simulink model "Quarter_Car_Model_Simulation"  (R2019a)
settings: Solver=VariableStepAuto  StartTime=0.0  StopTime=16  RelTol=1e-3
settings Model: Creator=Arun  LastModifiedBy=Arun

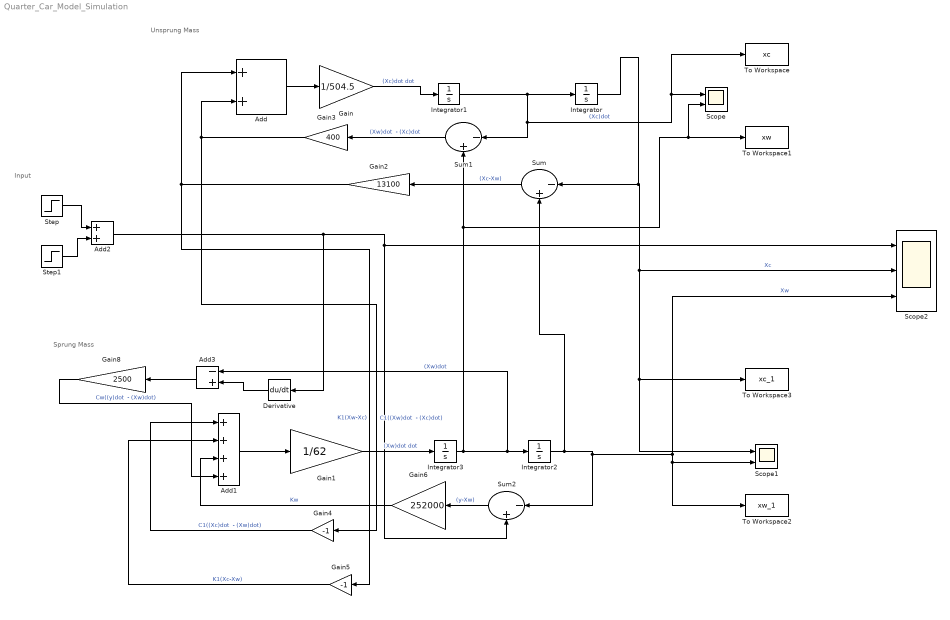
== system Quarter_Car_Model_Simulation ==
  note: Sprung Mass
  note: Unsprung Mass
  note: Input
  Add : Sum
  Add1 : Sum  Inputs=++++
  Add2 : Sum
  Add3 : Sum  Inputs=-+
  Derivative : Derivative
  Gain : Gain  Gain=1/504.5
  Gain1 : Gain  Gain=1/62
  Gain2 : Gain  Gain=13100
  Gain3 : Gain  Gain=400
  Gain4 : Gain  Gain=-1
  Gain5 : Gain  Gain=-1
  Gain6 : Gain  Gain=252000
  Gain8 : Gain  Gain=2500
  Integrator{,1..3} (4 alike) : Integrator
  Scope : Scope  NumInputPorts=2
  Scope1 : Scope  NumInputPorts=2
  Scope2 : Scope  NumInputPorts=3
  Step : Step  Time=3  After=10  SampleTime=0
  Step1 : Step  Time=5  After=-10  SampleTime=0
  Sum : Sum  Inputs=|-+
  Sum1 : Sum  Inputs=|-+
  Sum2 : Sum  Inputs=|-+
  To Workspace : ToWorkspace  VariableName=xc  SampleTime=1
  To Workspace1 : ToWorkspace  VariableName=xw  SaveFormat=Timeseries  SampleTime=1
  To Workspace2 : ToWorkspace  VariableName=xw_1  SaveFormat=Timeseries  SampleTime=1
  To Workspace3 : ToWorkspace  VariableName=xc_1  SampleTime=1
  wires:
  Integrator/1 -> To Workspace3/1, Scope1/1, Scope2/2, Sum/1  "Xc"
  Gain/1 -> Integrator1/1  "(Xc)dot dot"
  Integrator1/1 -> Integrator/1, Scope/1, To Workspace/1, Sum1/1  "(Xc)dot"
  Add/1 -> Gain/1
  Add1/1 -> Gain1/1
  Integrator3/1 -> Add3/1, Integrator2/1, To Workspace1/1, Scope/2, Sum1/2  "(Xw)dot"
  Gain1/1 -> Integrator3/1  "(Xw)dot dot"
  Integrator2/1 -> Sum2/1, To Workspace2/1, Scope1/2, Scope2/3, Sum/2  "Xw"
  Sum/1 -> Gain2/1  "(Xc-Xw)"
  Gain2/1 -> Gain5/1, Add/1  "K1(Xw-Xc)"
  Sum1/1 -> Gain3/1  "(Xw)dot  - (Xc)dot"
  Gain3/1 -> Gain4/1, Add/2  "C1((Xw)dot  - (Xc)dot)"
  Gain4/1 -> Add1/1  "C1((Xc)dot  - (Xw)dot)"
  Gain5/1 -> Add1/2  "K1(Xc-Xw)"
  Step/1 -> Add2/1
  Step1/1 -> Add2/2
  Add2/1 -> Scope2/1, Sum2/2, Derivative/1
  Sum2/1 -> Gain6/1  "(y-Xw)"
  Gain6/1 -> Add1/3  "Kw"
  Gain8/1 -> Add1/4  "Cw((y)dot  - (Xw)dot)"
  Add3/1 -> Gain8/1
  Derivative/1 -> Add3/2
